simulink model "DTSMC_Gao_TWMR_velocity"  (R2018b)
settings: Solver=VariableStepAuto  StartTime=0.0  StopTime=100  RelTol=1e-3
values from neighbouring files (symbols this model uses):
  c1 = c(1)    [DTSMC_Gao_TWMR_Position_param.m]    (also in DTSMC_Gao_TWMR_velocity_param.m)
libraries: simulink x1
settings Model: Creator=baleshwar  LastModifiedBy=baleshwar

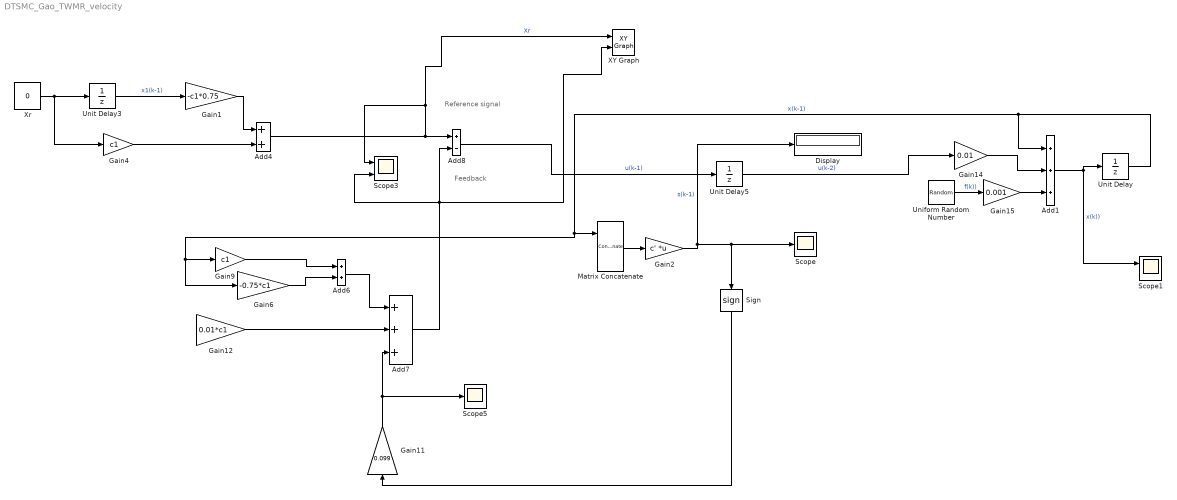
== system DTSMC_Gao_TWMR_velocity ==
  note: Feedback
  note: Reference signal
  Add1 : Sum  Inputs=+++
  Add4 : Sum
  Add6 : Sum
  Add7 : Sum  Inputs=+++
  Add8 : Sum  Inputs=+-
  Display : Display
  Gain1 : Gain  Gain=-c1*0.75
  Gain11 : Gain  Gain=0.099
  Gain12 : Gain  Gain=0.01*c1
  Gain14 : Gain  Gain=0.01
  Gain15 : Gain  Gain=0.001
  Gain2 : Gain  Gain=c'  Multiplication=Matrix(K*u)
  Gain4 : Gain  Gain=c1
  Gain6 : Gain  Gain=-0.75*c1
  Gain9 : Gain  Gain=c1
  Matrix Concatenate : Concatenate  Mode=Multidimensional array
  Scope : Scope
  Scope1 : Scope  NumInputPorts=2
  Scope3 : Scope  NumInputPorts=2
  Scope5 : Scope
  Sign : Signum
  Uniform Random Number : UniformRandomNumber  Minimum=-0.05  Maximum=0.05  SampleTime=0.01
  Unit Delay : UnitDelay  SampleTime=0.01
  Unit Delay3 : UnitDelay  SampleTime=0.1
  Unit Delay5 : UnitDelay  SampleTime=0.01
  XY Graph : simulink/Sinks/XY Graph  xmin=-inf  xmax=inf  ymin=-inf  ymax=inf  st=0.1
  Xr : Constant  Value=0  SampleTime=0.01
  wires:
  Add8/1 -> Unit Delay5/1  "u(k-1)"
  Gain12/1 -> Add7/2
  Uniform Random Number/1 -> Gain15/1  "f(k))"
  Gain2/1 -> Display/1, Scope/1, Sign/1  "s(k-1)"
  Xr/1 -> Unit Delay3/1, Gain4/1
  Gain6/1 -> Add6/2
  Gain1/1 -> Add4/1
  Unit Delay/1 -> Add1/1, Matrix Concatenate/1, Gain6/1, Gain9/1  "x(k-1)"
  Unit Delay3/1 -> Gain1/1  "x1(k-1)"
  Add7/1 -> XY Graph/2, Scope3/2, Add8/2
  Gain9/1 -> Add6/1
  Add6/1 -> Add7/1
  Sign/1 -> Gain11/1
  Add4/1 -> XY Graph/1, Scope3/1, Add8/1  "Xr"
  Gain11/1 -> Scope5/1, Add7/3
  Add1/1 -> Unit Delay/1, Scope1/1  "x(k))"
  Gain4/1 -> Add4/2
  Matrix Concatenate/1 -> Gain2/1
  Unit Delay5/1 -> Gain14/1  "u(k-2)"
  Gain14/1 -> Add1/2
  Gain15/1 -> Add1/3
